simulink model "simulation"  (Simulink 9.2)
settings: Solver=ode4  StartTime=0.0  StopTime=30  FixedStep=0.001  RelTol=1e-3  EnableMultiTasking=on
settings Model: Creator=lenovo  LastModifiedBy=lenovo  ExtModeTrigMode=oneshot  ExtModeArmWhenConnect=off
settings DataIOCC: LimitDataPoints=off  SignalLoggingName=sigsOut
settings OptimizationCC: BooleanDataType=off  LifeSpan=auto
settings DebuggingCC: SaveWithParameterizedLinksMsg=none  SignalResolutionControl=TryResolveAllWithWarning  MultiTaskDSMMsg=warning  MultiTaskCondExecSysMsg=none  FcnCallInpInsideContextMsg=error  StateNameClashWarn=none  SFUnexpectedBacktrackingDiag=error  SFNoUnconditionalDefaultTransitionDiag=error  SFExecutionAtInitializationDiag=warning
settings HardwareCC: TargetUnknown=on
settings SFSimCC: SimUseLocalCustomCode=on
settings RTWCC: RTWUseLocalCustomCode=on
settings CodeAppCC: StateflowObjectComments=off
settings GRTTargetCC: TargetLangStandard=C99 (ISO)  GeneratePreprocessorConditionals=Use local settings
settings ConfigComp: CovExternalEMLEnable=on

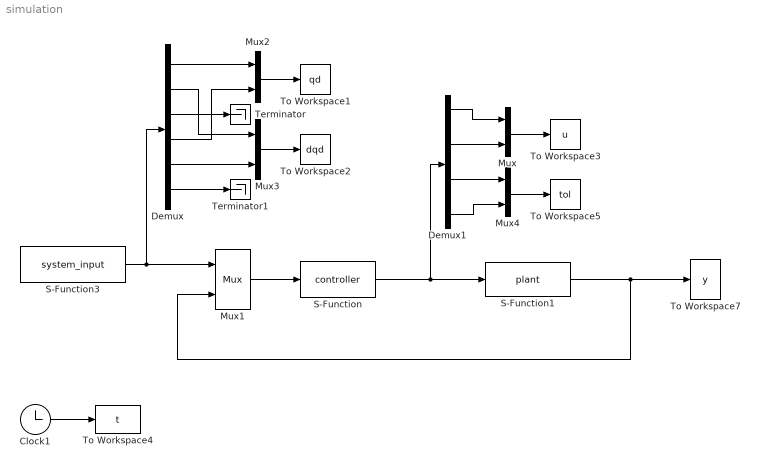
== system simulation ==
  Clock1 : Clock
  Demux : Demux  Outputs=6
  Demux1 : Demux
  Mux{,1..4} (5 alike) : Mux  Inputs=2
  S-Function : S-Function  FunctionName=controller  SFunctionDeploymentMode=off  EnableBusSupport=off
  S-Function1 : S-Function  FunctionName=plant  SFunctionDeploymentMode=off  EnableBusSupport=off
  S-Function3 : S-Function  FunctionName=system_input  SFunctionDeploymentMode=off  EnableBusSupport=off
  Terminator : Terminator
  Terminator1 : Terminator
  To Workspace1 : ToWorkspace  VariableName=qd  SampleTime=-1
  To Workspace2 : ToWorkspace  VariableName=dqd  SampleTime=-1
  To Workspace3 : ToWorkspace  VariableName=u  SampleTime=-1
  To Workspace4 : ToWorkspace  VariableName=t  SampleTime=-1
  To Workspace5 : ToWorkspace  VariableName=tol  SampleTime=-1
  To Workspace7 : ToWorkspace  VariableName=y  SampleTime=-1
  wires:
  S-Function/1 -> Demux1/1, S-Function1/1
  S-Function1/1 -> Mux1/2, To Workspace7/1
  Mux1/1 -> S-Function/1
  Mux2/1 -> To Workspace1/1
  S-Function3/1 -> Demux/1, Mux1/1
  Demux/1 -> Mux2/1
  Mux3/1 -> To Workspace2/1
  Demux/3 -> Terminator/1
  Demux/6 -> Terminator1/1
  Clock1/1 -> To Workspace4/1
  Demux1/1 -> Mux/1
  Demux1/2 -> Mux/2
  Mux/1 -> To Workspace3/1
  Mux4/1 -> To Workspace5/1
  Demux1/3 -> Mux4/1
  Demux1/4 -> Mux4/2
  Demux/5 -> Mux3/2
  Demux/4 -> Mux2/2
  Demux/2 -> Mux3/1
